simulink model "dcmotor_sim"  (R2023a)
settings: Solver=VariableStepAuto  StartTime=0.0  StopTime=3  MaxStep=1e-4  RelTol=1e-3
undefined symbols (not defined in the file or in its folder): k, kp, p
libraries: cstblocks x2
settings Model: Creator=Michael Peter  LastModifiedBy=Michael Peter

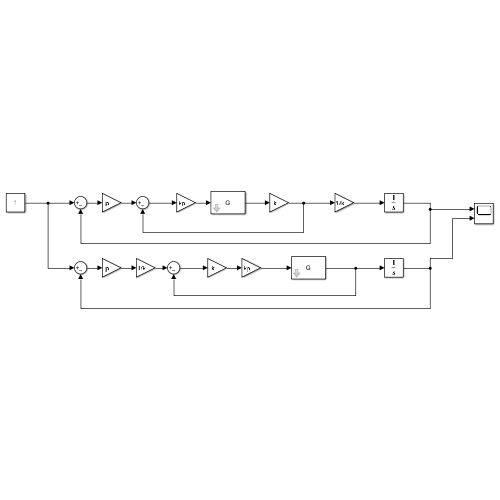
[thumbnail: Simulink's stored preview of the top-level diagram]
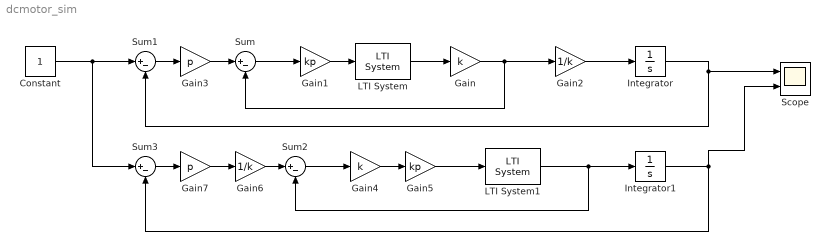
== system dcmotor_sim ==
  Constant : Constant
  Gain : Gain  Gain=k
  Gain1 : Gain  Gain=kp
  Gain2 : Gain  Gain=1/k
  Gain3 : Gain  Gain=p
  Gain4 : Gain  Gain=k
  Gain5 : Gain  Gain=kp
  Gain6 : Gain  Gain=1/k
  Gain7 : Gain  Gain=p
  Integrator : Integrator
  Integrator1 : Integrator
  LTI System : cstblocks/LTI System  sys=G  IC=[]
  LTI System1 : cstblocks/LTI System  sys=G  IC=[]
  Scope : Scope  NumInputPorts=2
  Sum{,1..3} (4 alike) : Sum  Inputs=|+-
  wires:
  LTI System/1 -> Gain/1
  Sum/1 -> Gain1/1
  Gain1/1 -> LTI System/1
  Gain/1 -> Gain2/1, Sum/2
  Gain2/1 -> Integrator/1
  Integrator/1 -> Sum1/2, Scope/1
  Sum1/1 -> Gain3/1
  Gain3/1 -> Sum/1
  Constant/1 -> Sum3/1, Sum1/1
  Sum3/1 -> Gain7/1
  Integrator1/1 -> Scope/2, Sum3/2
  LTI System1/1 -> Integrator1/1, Sum2/2
  Gain5/1 -> LTI System1/1
  Sum2/1 -> Gain4/1
  Gain4/1 -> Gain5/1
  Gain6/1 -> Sum2/1
  Gain7/1 -> Gain6/1
